simulink model "Final_openloop"  (R2024b)
settings: Solver=ode23s  StartTime=0.0  StopTime=150  RelTol=1e-3
(part 2 of 2)

== matlab function Final_openloop/MATLAB Function5 ==
  data: u input; y output
function y = Neutralization(u)

% inputs
Q=u(1);
C_X_S=u(2);
C_Dis=u(3);
C_Plasmid=u(4);
C_De=u(5);
C_Endo=u(6);
C_NaOH=u(7);
C_CH3CO2K=u(8);

% Reaction
Q_neutralization=Q*0.5;

y=zeros(1,8);
y(1) = (Q+Q_neutralization);                                %Q total
y(2) = (C_X_S*Q)/(Q+Q_neutralization);                      %C_X_F
y(3) = (C_Dis*Q)/(Q+Q_neutralization);                      %C_disruption_F
y(4) = (C_Plasmid*Q)/(Q+Q_neutralization);                  %C_plasmid_F
y(5) = (C_De*Q)/(Q+Q_neutralization);                       %C_denaturated_F
y(6) = (C_Endo*Q)/(Q+Q_neutralization);                     %C_endotoxin_F
y(7) = (C_NaOH*Q)/(Q+Q_neutralization);                     %C_NaOH_F
y(8) = (C_CH3CO2K*Q_neutralization)/(Q+Q_neutralization);   %C_CH3CO2K_F

== matlab function Final_openloop/UF-301 ==
  data: u input; y output
function y  = UF(u)

%input
C_pDNA=u(1);
C_lin_pDNA=u(2);
C_Impurities=u(3);
C_Enzyme=u(4);
Q_IN=u(5);
P=u(6);
A=u(7);

%% parameters for nanofiltration 

P_0 = 0.49; % referece pressure (kPa)
alpha_0=10.2*10^12; % reference.
n=0.5; % 
%A=0.1036; % membrane area (m^2)
eta_perm=1.0*10^-8; % Viscosity (kPa*s)
m_x_c=7.7*10^-3; % (kg)
R_m =1.26*10^12; % (1/m)

% Calculate alpha based on P_TM
alpha = alpha_0 * (P / P_0)^n;

% Calculate R_C
R_C = alpha * (m_x_c) / A;


dim=10;
y=zeros(dim,1);

 %% Rejection coefficients for different species
Rej=[0.01; 0.01; 0.01; -0.0250*P^4-0.0236*P^3+0.0927*P^2+0.4960*P+0.1979];


%% Output calculation

    y(1)=((P/(eta_perm * (R_m + R_C)))*A)*1000*3600;% Permeate flow (L/m^2/h)

    y(2)=Q_IN-y(1); % Retentate
    
%% Species balances for retentate stream (calculated based on inflow and rejection)
    y(3)=(Q_IN*C_pDNA)/(y(2)+y(1)*(1-Rej(1)));              % pDNA species balance retentate stream
    y(4)=(Q_IN*C_lin_pDNA)/(y(2)+y(1)*(1-Rej(2)));          % LinpDNA species balance retentate stream
    y(5)=(Q_IN*C_Impurities)/(y(2)+y(1)*(1-Rej(3)));        % Impurties species balance retentate stream
    y(6)=(Q_IN*C_Enzyme)/(y(2)+y(1)*(1-Rej(4)));            % Enzyme plasmid species balance retentate stream

%% Species concentrations in permeate stream (calculated based on rejection) 
    y(7)=y(3)*(1-Rej(1));                                   % pDNA concentration in permeate stream
    y(8)=y(4)*(1-Rej(2));                                   % LinpDNA concentration in permeate stream
    y(9)=y(5)*(1-Rej(3));                                   % Impurities concentration in permeate stream
    y(10)=y(6)*(1-Rej(4));                                  % Enzyme concentration in permeate stream

end

== matlab function Final_openloop/VSP-301 ==
  data: u input size=2; y output size=2
function y  = Pump(u)

%input
Q_C=u(1);
n=u(2);



y=zeros(2,1);

% output

y(1)=Q_C;
y(2)=((-0.085*Q_C^2 - 0.0000329*Q_C*n + 0.0000155555555555556*n^2)*(997*9.81))/10^5;


end

== matlab function Final_openloop/UF-401 ==
  data: u input; y output
function y = UF(u)
    % Input concentrations for each species in the feed stream
    C_mRNA = u(1);              % mRNA concentration (g/L)
    C_impurities = u(2);        % Impurities concentration (g/L)
    C_T7 = u(3);                % Ea T7 concentration (g/L)
    C_linpDNA = u(4);           % linpDNA concentration (g/L)
    C_cleancap = u(5);          % CleanCap concentration (g/L)
    C_magnesium = u(6);         % MgAcetate concentration (g/L)
    C_nucleo = u(7);            % Nucleotides concentration (g/L)
    C_degrade = u(8);           % Degrade concentration (g/L)
    C_Ea_DNase = u(9);          % DNase I concentration (g/L)
    Q_IN = u(10);               % Inflow rate (L/h)
    P = u(11);                  % Transmembrane pressure (kPa)
    A=u(12);

    %% Parameters for nanofiltration
    P_0 = 0.49;           % Reference pressure (kPa)
    alpha_0 = 10.2e12;    % Reference alpha
    n = 0.5;              % Pressure exponent
    eta_perm = 1.0e-8;    % Viscosity (kPa*s)
    m_x_c = 7.7e-3;       % (kg)
    R_m = 1.26e12;        % (1/m)

    % Calculate alpha based on P_TM
    alpha = alpha_0 * (P / P_0)^n;

    % Calculate R_C
    R_C = alpha * (m_x_c) / A;

    % Time and dimension parameters
    dim = 20;           % Number of outputs (8 species in both retentate and permeate)
    y = zeros(dim, 1);  % Initialize output vector

    %% Rejection coefficients for different species
    Rej = [-0.0250*P^4 - 0.0236*P^3 + 0.0927*P^2 + 0.4960*P + 0.1979; 0.50; -0.0250*P^4 - 0.0236*P^3 + 0.0927*P^2 + 0.4960*P + 0.1979; 0.01; -0.0250*P^4 - 0.0236*P^3 + 0.0927*P^2 + 0.4960*P + 0.1979; -0.0250*P^4 - 0.0236*P^3 + 0.0927*P^2 + 0.4960*P + 0.1979; 0.01; 0.01;0.01];
   
    %% Output calculations
    % Permeate flow rate (L/m^2/h)
    y(1) = (P / (eta_perm * (R_m + R_C))) * A * 1000 * 3600;            % Permeate flow (L/m^2/h)
    y(2) = Q_IN - y(1);                                                 % Retentate flow
    
    % Species balances for retentate stream (calculated based on inflow and rejection)
   y(3) = (Q_IN * C_mRNA) / (y(2) + y(1) * (1 - Rej(1)));               % mRNA concentration in retentate
    y(4) = (Q_IN * C_impurities) / (y(2) + y(1) * (1 - Rej(2)));        % Assumed 50% impurities futher in the system.Impurities concentration in retentate
    y(5) = (Q_IN * C_T7) / (y(2) + y(1) * (1 - Rej(3)));                % Ea T7 concentration in retentate
    y(6) = (Q_IN * C_linpDNA) / (y(2) + y(1) * (1 - Rej(4)));           % linpDNA (DNA template) concentration in retentate
    y(7) = (Q_IN * C_cleancap) / (y(2) + y(1) * (1 - Rej(5)));          % CleanCap concentration in retentate
    y(8) = (Q_IN * C_magnesium) / (y(2) + y(1) * (1 - Rej(6)));         % MgAcetate concentration in retentate
    y(9) = (Q_IN * C_nucleo) / (y(2) + y(1) * (1 - Rej(7)));            % Nucleotides concentration in retentate
    y(10) = (Q_IN * C_degrade) / (y(2) + y(1) * (1 - Rej(8)));          % Degrade concentration in retentate
    y(11) = (Q_IN * C_Ea_DNase) / (y(2) + y(1) * (1 - Rej(9)));         % DNase I concentration in retentatem

    %% Species concentrations in permeate stream (calculated based on rejection)
    y(12) = y(3) * (1 - Rej(1));  % mRNA concentration in permeate
    y(13) = y(4) * (1 - Rej(2));  % Impurities concentration in permeate
    y(14) = y(5) * (1 - Rej(3));  % Ea T7 concentration in permeate
    y(15) = y(6) * (1 - Rej(4));  % linpDNA (DNA template) concentration in permeate
    y(16) = y(7) * (1 - Rej(5));  % CleanCap concentration in permeate
    y(17) = y(8) * (1 - Rej(6));  % MgAcetate concentration in permeate
    y(18) = y(9) * (1 - Rej(7));  % Nucleotides concentration in permeate
    y(19) = y(10) * (1 - Rej(8)); % Degrade concentration in permeate
    y(20) = y(11) * (1 - Rej(9)); % DNase concentration in permeate
 


end

== matlab function Final_openloop/VSP-401 ==
  data: u input size=2; y output size=2
function y  = Pump(u)

%input
Q_C=u(1);
n=u(2);



y=zeros(2,1);

% output

y(1)=Q_C;
y(2)=((-0.085*Q_C^2 - 0.0000329*Q_C*n + 0.0000155555555555556*n^2)*(997*9.81))/10^5;


end
